simulink model "simulacao_sis2aord"  (R2018a)
settings: Solver=FixedStepAuto  StartTime=0.0  StopTime=ns  FixedStep=1  RelTol=1e-3
values from neighbouring files (symbols this model uses):
  a = exp(-Ts/tau)    [exempl3_1.m]    (also in vrft_ex31_v2.m = exp(-1/tau*Ts); vrft_ex31_v3.m = exp(-1/tau*Ts); vrft_ex31_v4.m = exp(-1/tau*Ts); vrft_pid_mr1ao.m = exp(-1/tau*Ts))
  C1 = tf(theta1(1:3)', [1 -theta1(4:end)'],Ts)    [exempl3_1.m]
  C2 = tf(theta2(1:3)', [1 -theta2(4)' 0],Ts)    [exempl3_1.m]
  C3 = Kp + Ki*z/(z-1) + Kd*(z-1)/z    [exempl3_1.m]
  C4 = tf(theta4_cls(1:3)', [1 -theta4_cls(4)' 0],Ts)    [exempl3_1.m]
  distAmp = 0.5    [exempl3_1.m]
  distTime = 75    [exempl3_1.m]
  G = (b1*z + b2)/(z^2-a1*z-a2)    [contr_ideal.m]    (also in exempl3_1.m = tf([0 rho(3:4)'],[1 -rho(1:2)'],Ts))
  tau = 5    [contr_ideal.m]    (also in exempl3_1.m)
  Ts = 1    [contr_ideal.m]    (also in exempl3_1.m; vrft_ex31_v2.m = h; vrft_ex31_v3.m = h; vrft_ex31_v4.m = h)
settings Model: Creator=joao  LastModifiedBy=joao

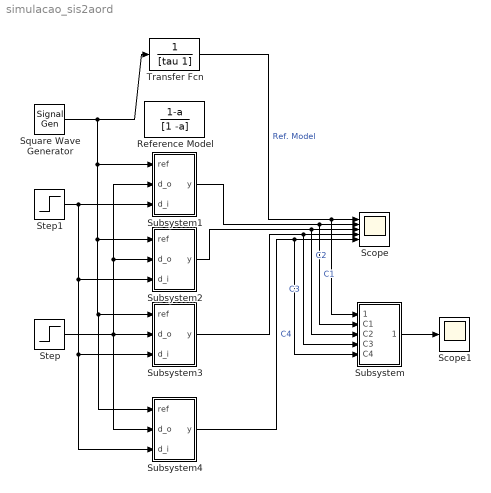
== system simulacao_sis2aord ==
  Reference Model : DiscreteTransferFcn  Numerator=1-a  Denominator=[1 -a]
  Scope : Scope  NumInputPorts=5
  Scope1 : Scope
  Square Wave Generator : SignalGenerator  WaveForm=square  Frequency=1/100
  Step : Step  Time=distTime  After=distAmp  SampleTime=Ts
  Step1 : Step  Time=distTime  After=0  SampleTime=Ts
  Subsystem : Subsystem
  Subsystem1 : Subsystem
  Subsystem2 : Subsystem
  Subsystem3 : Subsystem
  Subsystem4 : Subsystem
  Transfer Fcn : TransferFcn  Denominator=[tau 1]
  wires:
  Square Wave Generator/1 -> Transfer Fcn/1, Subsystem4/1(ref), Subsystem3/1(ref), Subsystem2/1(ref), Subsystem1/1(ref)
  Step/1 -> Subsystem4/2(d_o), Subsystem3/2(d_o), Subsystem2/2(d_o), Subsystem1/2(d_o)
  Transfer Fcn/1 -> Subsystem/1(RM), Scope/1  "Ref. Model"
  Subsystem1/1(y) -> Subsystem/2(C1), Scope/2  "C1"
  Subsystem3/1(y) -> Subsystem/4(C3), Scope/4  "C3"
  Step1/1 -> Subsystem4/3(d_i), Subsystem3/3(d_i), Subsystem2/3(d_i), Subsystem1/3(d_i)
  Subsystem2/1(y) -> Subsystem/3(C2), Scope/3  "C2"
  Subsystem4/1(y) -> Subsystem/5(C4), Scope/5  "C4"
  Subsystem/1(error) -> Scope1/1

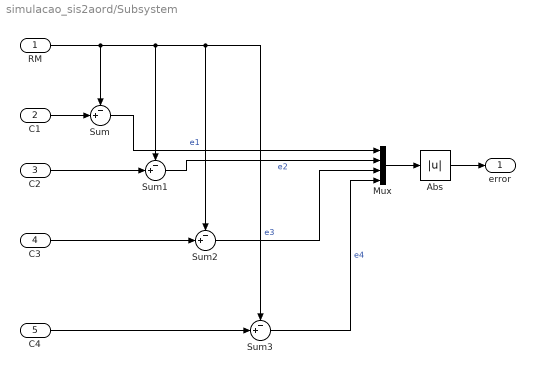
== system simulacao_sis2aord/Subsystem ==
  RM : Inport
  C1 : Inport  Port=2
  C2 : Inport  Port=3
  C3 : Inport  Port=4
  C4 : Inport  Port=5
  Abs : Abs
  Mux : Mux
  Sum{,1..3} (4 alike) : Sum  Inputs=-+|
  error : Outport
  wires:
  C1/1 -> Sum/2
  C2/1 -> Sum1/2
  C3/1 -> Sum2/2
  C4/1 -> Sum3/2
  RM/1 -> Sum3/1, Sum2/1, Sum1/1, Sum/1
  Sum/1 -> Mux/1  "e1"
  Sum1/1 -> Mux/2  "e2"
  Sum2/1 -> Mux/3  "e3"
  Sum3/1 -> Mux/4  "e4"
  Mux/1 -> Abs/1
  Abs/1 -> error/1

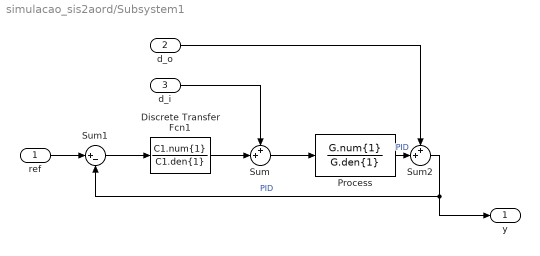
== system simulacao_sis2aord/Subsystem1 ==
  ref : Inport
  d_o : Inport  Port=2
  d_i : Inport  Port=3
  Discrete Transfer Fcn1 : DiscreteTransferFcn  Numerator=C1.num{1}  Denominator=C1.den{1}
  Process : DiscreteTransferFcn  Numerator=G.num{1}  Denominator=G.den{1}
  Sum : Sum  Inputs=++|
  Sum1 : Sum  Inputs=|+-
  Sum2 : Sum  Inputs=++|
  y : Outport
  wires:
  d_o/1 -> Sum2/1
  Discrete Transfer Fcn1/1 -> Sum/2
  Sum2/1 -> Sum1/2, y/1  "PID"
  Sum1/1 -> Discrete Transfer Fcn1/1
  ref/1 -> Sum1/1
  Sum/1 -> Process/1
  Process/1 -> Sum2/2  "PID"
  d_i/1 -> Sum/1

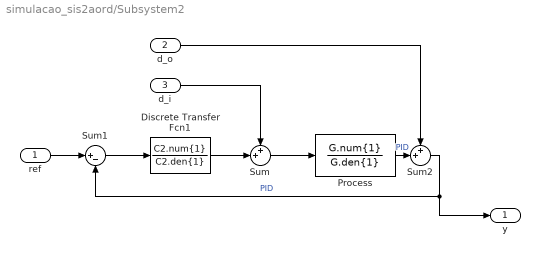
== system simulacao_sis2aord/Subsystem2 ==
  ref : Inport
  d_o : Inport  Port=2
  d_i : Inport  Port=3
  Discrete Transfer Fcn1 : DiscreteTransferFcn  Numerator=C2.num{1}  Denominator=C2.den{1}
  Process : DiscreteTransferFcn  Numerator=G.num{1}  Denominator=G.den{1}
  Sum : Sum  Inputs=++|
  Sum1 : Sum  Inputs=|+-
  Sum2 : Sum  Inputs=++|
  y : Outport
  wires:
  d_i/1 -> Sum/1
  Process/1 -> Sum2/2  "PID"
  Sum/1 -> Process/1
  ref/1 -> Sum1/1
  Sum1/1 -> Discrete Transfer Fcn1/1
  Sum2/1 -> y/1, Sum1/2  "PID"
  Discrete Transfer Fcn1/1 -> Sum/2
  d_o/1 -> Sum2/1

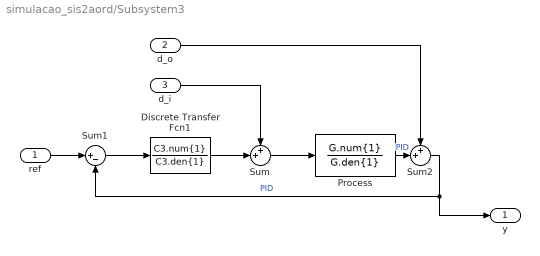
== system simulacao_sis2aord/Subsystem3 ==
  ref : Inport
  d_o : Inport  Port=2
  d_i : Inport  Port=3
  Discrete Transfer Fcn1 : DiscreteTransferFcn  Numerator=C3.num{1}  Denominator=C3.den{1}
  Process : DiscreteTransferFcn  Numerator=G.num{1}  Denominator=G.den{1}
  Sum : Sum  Inputs=++|
  Sum1 : Sum  Inputs=|+-
  Sum2 : Sum  Inputs=++|
  y : Outport
  wires:
  d_o/1 -> Sum2/1
  Discrete Transfer Fcn1/1 -> Sum/2
  Sum2/1 -> Sum1/2, y/1  "PID"
  Sum1/1 -> Discrete Transfer Fcn1/1
  ref/1 -> Sum1/1
  Sum/1 -> Process/1
  Process/1 -> Sum2/2  "PID"
  d_i/1 -> Sum/1

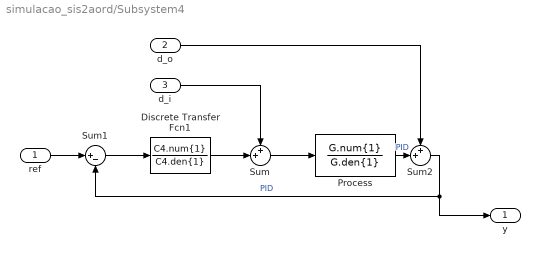
== system simulacao_sis2aord/Subsystem4 ==
  ref : Inport
  d_o : Inport  Port=2
  d_i : Inport  Port=3
  Discrete Transfer Fcn1 : DiscreteTransferFcn  Numerator=C4.num{1}  Denominator=C4.den{1}
  Process : DiscreteTransferFcn  Numerator=G.num{1}  Denominator=G.den{1}
  Sum : Sum  Inputs=++|
  Sum1 : Sum  Inputs=|+-
  Sum2 : Sum  Inputs=++|
  y : Outport
  wires:
  d_i/1 -> Sum/1
  Process/1 -> Sum2/2  "PID"
  Sum/1 -> Process/1
  ref/1 -> Sum1/1
  Sum1/1 -> Discrete Transfer Fcn1/1
  Sum2/1 -> y/1, Sum1/2  "PID"
  Discrete Transfer Fcn1/1 -> Sum/2
  d_o/1 -> Sum2/1
